simulink model "fullmodel"  (R2018a)
settings: Solver=VariableStepAuto  StartTime=0.0  StopTime=15  RelTol=1e-3
undefined symbols (not defined in the file): duty
libraries: powerlib x19, powerlib_meascontrol x2, pePowerMeasurement x1, simulink x1
settings Model: Creator=DELL  LastModifiedBy=DELL

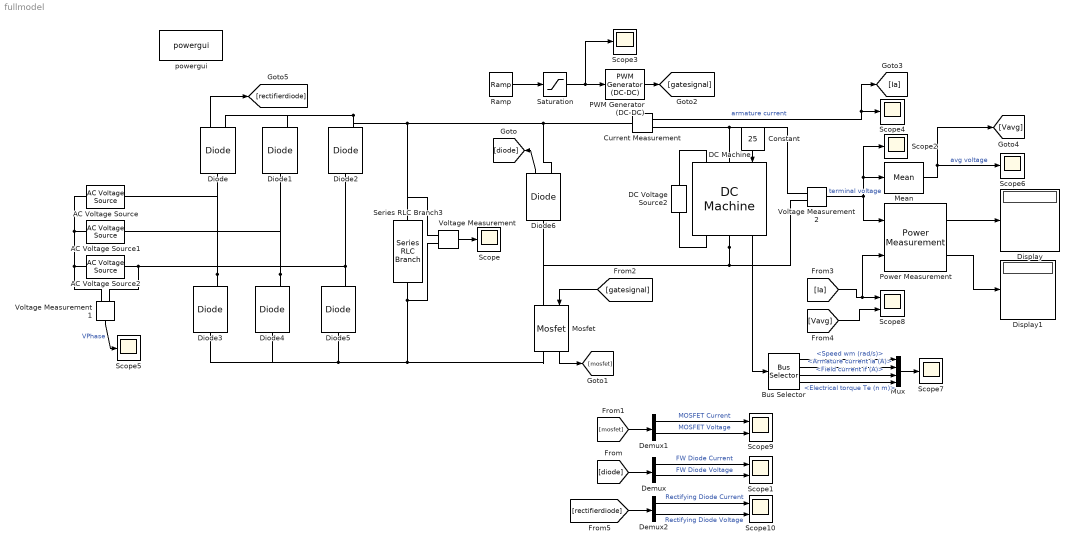
== system fullmodel ==
  AC Voltage Source : powerlib/Electrical Sources/AC Voltage Source  Amplitude=100*sqrt(2)  Phase=0  Frequency=50  SampleTime=0  Measurements=None  BusType=swing  Pref=10e3  Qref=0  Qmin=-inf  Qmax=+inf
  AC Voltage Source1 : powerlib/Electrical Sources/AC Voltage Source  Amplitude=100*sqrt(2)  Phase=-120  Frequency=50  SampleTime=0  Measurements=None  BusType=swing  Pref=10e3  Qref=0  Qmin=-inf  Qmax=+inf
  AC Voltage Source2 : powerlib/Electrical Sources/AC Voltage Source  Amplitude=100*sqrt(2)  Phase=120  Frequency=50  SampleTime=0  Measurements=None  BusType=swing  Pref=10e3  Qref=0  Qmin=-inf  Qmax=+inf
  Bus Selector : BusSelector  OutputSignals=Speed wm (rad/s),Armature current ia (A),Field current if (A),Electrical torque Te (n m)
  Constant : Constant  Value=25
  Current Measurement : powerlib/Measurements/Current Measurement  PhasorSimulation=off  OutputType=Complex  PSBequivalent=0
  DC Machine : powerlib/Machines/DC Machine  PresetModel=No  MechanicalLoad=Torque TL  FieldType=Wound  ShowDetailedParameters=on  MeasurementBus=off  RLa="[ 1.07  0.0245]"  RLf="[ 210  23]"  Laf=1.8  MachineConstant=Torque constant (N.m/A)  Ke=1.8  Kt=1.8  J=1  Bm=0  Tf=0  w0=1  Ifinit=1  TsPowergui=0  TsBlock=-1
  DC Voltage Source2 : powerlib/Electrical Sources/DC Voltage Source  Amplitude=220  Measurements=None
  Demux : Demux  Outputs=2
  Demux1 : Demux  Outputs=2
  Demux2 : Demux  Outputs=2
  Diode{,1..5} (6 alike) : powerlib/Power Electronics/Diode  Ron=0  Lon=0  Vf=0  IC=0  UseSnubber=0  Rs=inf  Cs=0  Measurements=on
  Diode6 : powerlib/Power Electronics/Diode  Ron=0.001  Lon=0  Vf=1.5  IC=0  UseSnubber=off  Rs=inf  Cs=0  Measurements=on
  Display : Display
  Display1 : Display
  Mean : powerlib_meascontrol/Measurements/Mean  Freq=60  Vinit=0  Ts=0
  Mosfet : powerlib/Power Electronics/Mosfet  Ron=0.085  Lon=0  Rd=0.01  Vfd=0  IC=0  Rs=1e5  Cs=inf  Measurements=on
  Mux : Mux
  PWM Generator (DC-DC) : powerlib_meascontrol/Pulse & Signal Generators/PWM Generator (DC-DC)  Fsw=20000  Ts=0
  Power Measurement : pePowerMeasurement/Power Measurement  OverrideUsingVariant=Continuous  F=60  K=[0 1 2 3]  Ts=0
  Ramp : simulink/Sources/Ramp  slope=duty/10  start=0  InitialOutput=0.9
  Saturation : Saturate  UpperLimit=0.9  LowerLimit=0  ZeroCross=off
  Scope{,2..7} (7 alike) : Scope
  Scope{1,8..10} (4 alike) : Scope  NumInputPorts=2
  Series RLC Branch3 : powerlib/Elements/Series RLC Branch  LConnTagsString=__new0  RConnTagsString=__new0  BranchType=C  Resistance=0.0001  Inductance=1e-3  SetiL0=off  InitialCurrent=0  Capacitance=1000e-6  Setx0=off  InitialVoltage=0  Measurements=None
  Voltage Measurement : powerlib/Measurements/Voltage Measurement  PhasorSimulation=off  OutputType=Complex  PSBequivalent=0
  Voltage Measurement1 : powerlib/Measurements/Voltage Measurement  PhasorSimulation=off  OutputType=Complex  PSBequivalent=0
  Voltage Measurement2 : powerlib/Measurements/Voltage Measurement  PhasorSimulation=off  OutputType=Complex  PSBequivalent=0
  powergui : powerlib/powergui  Priority=1  SimulationMode=Continuous  SampleTime=50e-6  frequency=60  Iterations=50  frequencyindice=0  Pbase=100e6  ErrMax=1e-4  UnitsV=kV  UnitsW=MW  buscounter=0  FunctionMessages=off  echomessages=off  EnableUseOfTLC=off  CurrentSourceSwitches=off  DisableSnubberDevices=off  DisableRonSwitches=off  DisableVfSwitches=off  DisplayEquations=off  SolverType=Tustin/Backward Euler (TBE)  Interpol=off  ExternalGateDelay=off  methode=off  Ts=100  x0status=blocks  SPID=on  SwTol=0  HookPort=off  RestoreLinks=warning  ResistiveCurrentMeasurement=off  Frange=[0:2:500]  Ylog=off  Xlog=on  ShowGrid=off  save=off  variable=ZData  structure=0  ZoomFFT=off  StartTime=0.0  cycles=1  DisplayStyle=1  fundamental=60  FreqAxis=off  MaxFrequency=1000  frequencyindicesteady=1  RmsSteady=1  display=off
  wires:
  Voltage Measurement/1 -> Scope/1
  Voltage Measurement1/1 -> Scope5/1  "VPhase"
  DC Machine/1 -> Bus Selector/1
  Bus Selector/1 -> Mux/1  "<Speed wm (rad/s)>"
  [mosfet] -> Demux1/1
  Demux/1 -> Scope1/1  "FW Diode Current"
  Bus Selector/4 -> Mux/4  "<Electrical torque Te (n m)>"
  Demux1/2 -> Scope9/2  "MOSFET Voltage"
  Saturation/1 -> Scope3/1, PWM Generator (DC-DC)/1
  [Vavg] -> Scope8/2
  PWM Generator (DC-DC)/1 -> [gatesignal]
  Power Measurement/1 -> Display/1
  Current Measurement/1 -> Scope4/1, [Ia]  "armature current"
  Ramp/1 -> Saturation/1
  Mosfet/1 -> [mosfet]
  Constant/1 -> DC Machine/1
  Demux1/1 -> Scope9/1  "MOSFET Current"
  Mean/1 -> Scope6/1, [Vavg]  "avg voltage"
  [gatesignal] -> Mosfet/1
  [Ia] -> Scope8/1, Power Measurement/2
  Bus Selector/3 -> Mux/3  "<Field current if (A)>"
  Demux/2 -> Scope1/2  "FW Diode Voltage"
  Diode6/1 -> [diode]
  Bus Selector/2 -> Mux/2  "<Armature current ia (A)>"
  Voltage Measurement2/1 -> Power Measurement/1, Scope2/1, Mean/1  "terminal voltage"
  [diode] -> Demux/1
  Power Measurement/2 -> Display1/1
  Mux/1 -> Scope7/1
  Diode/1 -> [rectifierdiode]
  [rectifierdiode] -> Demux2/1
  Demux2/2 -> Scope10/2  "Rectifying Diode Voltage"
  Demux2/1 -> Scope10/1  "Rectifying Diode Current"
  connections:
  AC Voltage Source2/RConn1 -- Diode2/LConn1 -- Diode5/RConn1 -- Voltage Measurement1/LConn1
  Diode4/RConn1 -- Diode1/LConn1 -- AC Voltage Source1/RConn1
  AC Voltage Source1/LConn1 -- AC Voltage Source/LConn1 -- Voltage Measurement1/LConn2 -- AC Voltage Source2/LConn1
  Diode3/RConn1 -- Diode/LConn1 -- AC Voltage Source/RConn1
  Current Measurement/LConn1 -- Diode6/RConn1 -- Voltage Measurement/LConn1 -- Series RLC Branch3/LConn1 -- Diode/RConn1 -- Diode1/RConn1 -- Diode2/RConn1
  Diode5/LConn1 -- Diode4/LConn1 -- Diode3/LConn1 -- Mosfet/RConn1 -- Voltage Measurement/LConn2 -- Series RLC Branch3/RConn1
  Current Measurement/RConn1 -- Voltage Measurement2/LConn1 -- DC Machine/LConn1
  DC Machine/RConn1 -- Voltage Measurement2/LConn2 -- Mosfet/LConn1 -- Diode6/LConn1
  DC Voltage Source2/RConn1 -- DC Machine/LConn2
  DC Voltage Source2/LConn1 -- DC Machine/RConn2
